simulink model "Lab1_Model3"  (R2021b)
settings: Solver=VariableStepAuto  StartTime=0.0  StopTime=10  RelTol=1e-3
libraries: cstblocks x2
settings Model: Creator=sarth  LastModifiedBy=sarth

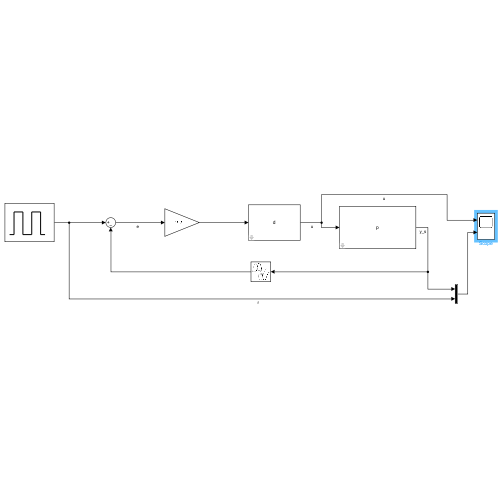
[thumbnail: Simulink's stored preview of the top-level diagram]
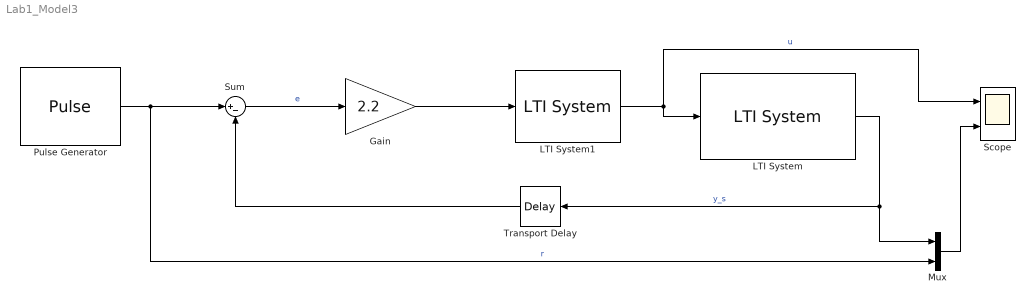
== system Lab1_Model3 ==
  Gain : Gain  Gain=2.2
  LTI System : cstblocks/LTI System  sys=p  IC=[]
  LTI System1 : cstblocks/LTI System  sys=d  IC=[]
  Mux : Mux  Inputs=2
  Pulse Generator : DiscretePulseGenerator  PulseType=Time based  Period=10  PulseWidth=50
  Scope : Scope  NumInputPorts=2
  Sum : Sum  Inputs=|+-
  Transport Delay : TransportDelay  DelayTime=0.0238
  wires:
  Sum/1 -> Gain/1  "e"
  Gain/1 -> LTI System1/1
  Mux/1 -> Scope/2
  Pulse Generator/1 -> Mux/2, Sum/1  "r"
  LTI System1/1 -> LTI System/1, Scope/1  "u"
  LTI System/1 -> Mux/1, Transport Delay/1  "y_s"
  Transport Delay/1 -> Sum/2
